simulink model "slip_ratio"  (R2015a)
settings: Solver=ode3  StartTime=0  StopTime=5  RelTol=1e-3
settings Model: Creator=BML  LastModifiedBy=BML
settings SolverCC: AutoInsertRateTranBlk=on

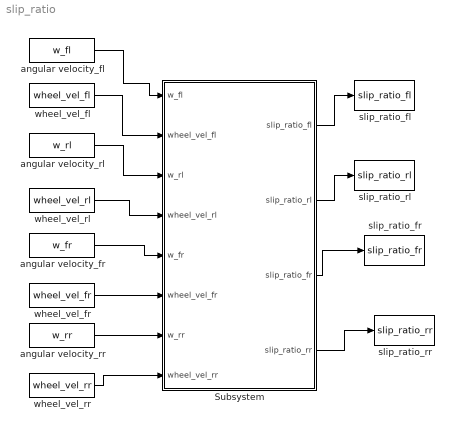
== system slip_ratio ==
  Subsystem : Subsystem
  angular velocity_fl : FromWorkspace  VariableName=w_fl  SampleTime=0
  angular velocity_fr : FromWorkspace  VariableName=w_fr  SampleTime=0
  angular velocity_rl : FromWorkspace  VariableName=w_rl  SampleTime=0
  angular velocity_rr : FromWorkspace  VariableName=w_rr  SampleTime=0
  slip_ratio_fl : ToWorkspace  VariableName=slip_ratio_fl  SaveFormat=Timeseries
  slip_ratio_fr : ToWorkspace  VariableName=slip_ratio_fr  SaveFormat=Timeseries
  slip_ratio_rl : ToWorkspace  VariableName=slip_ratio_rl  SaveFormat=Timeseries
  slip_ratio_rr : ToWorkspace  VariableName=slip_ratio_rr  SaveFormat=Timeseries
  wheel_vel_fl : FromWorkspace  VariableName=wheel_vel_fl  SampleTime=0
  wheel_vel_fr : FromWorkspace  VariableName=wheel_vel_fr  SampleTime=0
  wheel_vel_rl : FromWorkspace  VariableName=wheel_vel_rl  SampleTime=0
  wheel_vel_rr : FromWorkspace  VariableName=wheel_vel_rr  SampleTime=0
  wires:
  angular velocity_fl/1 -> Subsystem/1(w_fl)
  angular velocity_rl/1 -> Subsystem/3(w_rl)
  angular velocity_fr/1 -> Subsystem/5(w_fr)
  wheel_vel_fr/1 -> Subsystem/6(wheel_vel_fr)
  angular velocity_rr/1 -> Subsystem/7(w_rr)
  wheel_vel_rr/1 -> Subsystem/8(wheel_vel_rr)
  Subsystem/1(slip_ratio_fl) -> slip_ratio_fl/1
  Subsystem/2(slip_ratio_rl) -> slip_ratio_rl/1
  Subsystem/3(slip_ratio_fr) -> slip_ratio_fr/1
  Subsystem/4(slip_ratio_rr) -> slip_ratio_rr/1
  wheel_vel_fl/1 -> Subsystem/2(wheel_vel_fl)
  wheel_vel_rl/1 -> Subsystem/4(wheel_vel_rl)

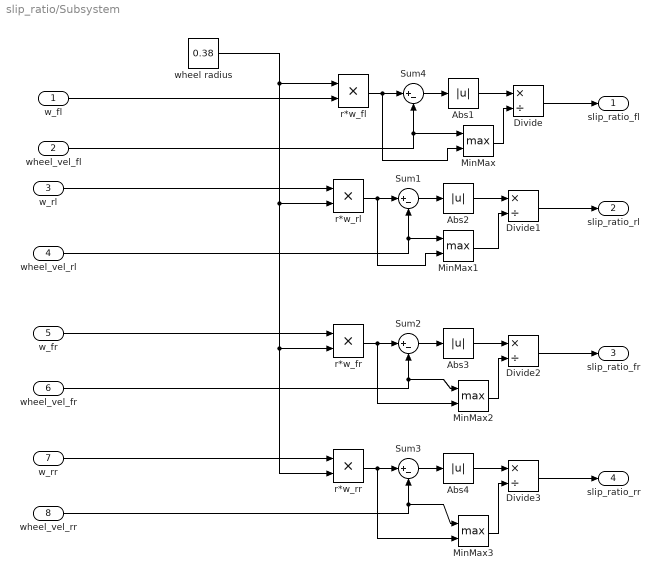
== system slip_ratio/Subsystem ==
  w_fl : Inport
  wheel_vel_fl : Inport  Port=2
  w_rl : Inport  Port=3
  wheel_vel_rl : Inport  Port=4
  w_fr : Inport  Port=5
  wheel_vel_fr : Inport  Port=6
  w_rr : Inport  Port=7
  wheel_vel_rr : Inport  Port=8
  Abs{1..4} (4 alike) : Abs
  Divide{,1..3} (4 alike) : Product  Inputs=*/
  MinMax{,1..3} (4 alike) : MinMax  Function=max  Inputs=2
  Sum{1..4} (4 alike) : Sum  Inputs=|+-
  r*w_fl : Product  Inputs=**
  r*w_fr : Product  Inputs=**
  r*w_rl : Product  Inputs=**
  r*w_rr : Product  Inputs=**
  wheel radius : Constant  Value=0.38
  slip_ratio_fl : Outport
  slip_ratio_rl : Outport  Port=2
  slip_ratio_fr : Outport  Port=3
  slip_ratio_rr : Outport  Port=4
  wires:
  w_fl/1 -> r*w_fl/2
  r*w_fl/1 -> MinMax/2, Sum4/1
  wheel radius/1 -> r*w_fl/1, r*w_rl/2, r*w_rr/2, r*w_fr/2
  wheel_vel_fl/1 -> Sum4/2, MinMax/1
  Sum4/1 -> Abs1/1
  Abs1/1 -> Divide/1
  MinMax/1 -> Divide/2
  Divide/1 -> slip_ratio_fl/1
  r*w_rl/1 -> MinMax1/2, Sum1/1
  wheel_vel_rl/1 -> Sum1/2, MinMax1/1
  Sum1/1 -> Abs2/1
  Abs2/1 -> Divide1/1
  MinMax1/1 -> Divide1/2
  Divide1/1 -> slip_ratio_rl/1
  w_rl/1 -> r*w_rl/1
  r*w_fr/1 -> MinMax2/2, Sum2/1
  wheel_vel_fr/1 -> MinMax2/1, Sum2/2
  Sum2/1 -> Abs3/1
  Abs3/1 -> Divide2/1
  MinMax2/1 -> Divide2/2
  Divide2/1 -> slip_ratio_fr/1
  w_fr/1 -> r*w_fr/1
  r*w_rr/1 -> MinMax3/2, Sum3/1
  wheel_vel_rr/1 -> MinMax3/1, Sum3/2
  Sum3/1 -> Abs4/1
  Abs4/1 -> Divide3/1
  MinMax3/1 -> Divide3/2
  Divide3/1 -> slip_ratio_rr/1
  w_rr/1 -> r*w_rr/1
